simulink model "ModelMotorDiscreto"  (R2012b)
settings: Solver=ode4  StartTime=0.0  StopTime=15  FixedStep=1e-4  RelTol=1e-3
undefined symbols (not defined in the file or in its folder): C2t
libraries: simulink x2
settings Model: Creator=Augusto  LastModifiedBy=Augusto

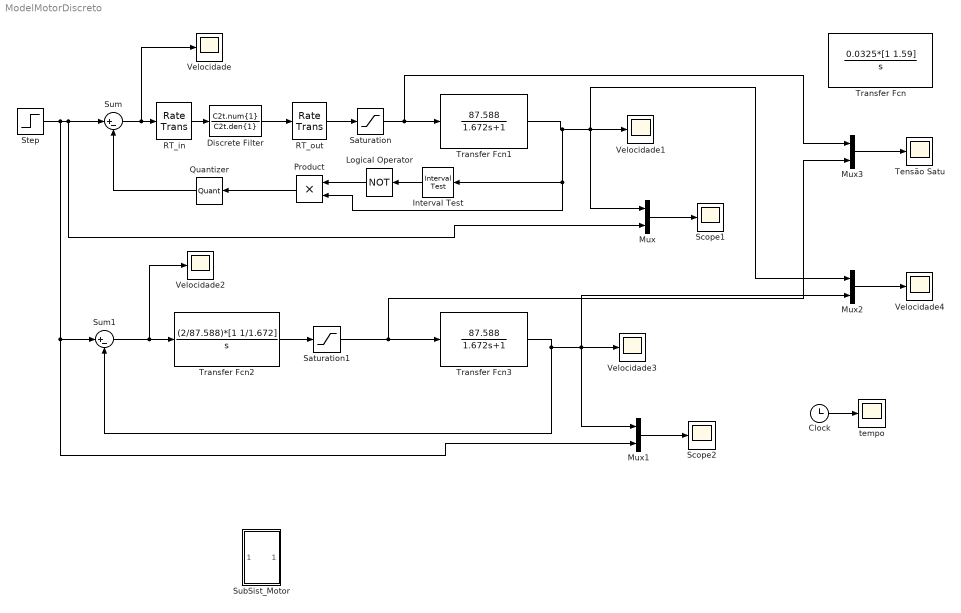
== system ModelMotorDiscreto ==
  Clock : Clock
  Discrete Filter : DiscreteFilter  Numerator=C2t.num{1}  Denominator=C2t.den{1}  SampleTime=C2t.Ts
  Interval Test : simulink/Logic and Bit Operations/Interval Test  IntervalClosedRight=on  uplimit=60*pi/30  IntervalClosedLeft=on  lowlimit=-60*pi/30  OutDataTypeStr=boolean
  Logical Operator : Logic  Operator=NOT  IconShape=distinctive  AllPortsSameDT=off  OutDataTypeStr=boolean
  Mux{,1..3} (4 alike) : Mux  Inputs=2
  Product : Product  RndMeth=Zero
  Quantizer : Quantizer  QuantizationInterval=100*pi/30
  RT_in : RateTransition  OutPortSampleTime=C2t.Ts
  RT_out : RateTransition  OutPortSampleTime=1e-4
  Saturation : Saturate  UpperLimit=11.4  LowerLimit=-11.4
  Saturation1 : Saturate  UpperLimit=11.4  LowerLimit=-11.4
  Scope1 : Scope
  Scope2 : Scope
      settings: YMin=628  YMax=628  SaveName=ScopeData3
  Step : Step  Time=100  Before=600  After=-628  SampleTime=0
  SubSist_Motor : Subsystem
  Sum : Sum  Inputs=|+-
  Sum1 : Sum  Inputs=|+-
  Tensão Satu : Scope
      settings: SaveName=ScopeData9
  Transfer Fcn : TransferFcn  Numerator=0.0325*[1 1.59]  Denominator=[1 0]
  Transfer Fcn1 : TransferFcn  Numerator=[87.588]  Denominator=[1.672 1]
  Transfer Fcn2 : TransferFcn  Numerator=(2/87.588)*[1 1/1.672]  Denominator=[1 0]
  Transfer Fcn3 : TransferFcn  Numerator=[87.588]  Denominator=[1.672 1]
  Velocidade{,1..4} (5 alike) : Scope
      Velocidade1 settings: SaveName=ScopeData2
      Velocidade2 settings: SaveName=ScopeData6
      Velocidade3 settings: SaveName=ScopeData7
      Velocidade4 settings: TimeRange=15  YMin=0  YMax=800  SaveName=ScopeData8
  tempo : Scope
      settings: Tag=Tempo  SaveName=ScopeData10
  wires:
  Mux/1 -> Scope1/1
  Sum/1 -> RT_in/1, Velocidade/1
  RT_out/1 -> Saturation/1
  Mux1/1 -> Scope2/1
  Sum1/1 -> Velocidade2/1, Transfer Fcn2/1
  Transfer Fcn2/1 -> Saturation1/1
  Transfer Fcn3/1 -> Sum1/2, Mux2/2, Mux1/1, Velocidade3/1
  Step/1 -> Sum1/1, Mux1/2, Sum/1, Mux/2
  Mux2/1 -> Velocidade4/1
  Saturation/1 -> Mux3/1, Transfer Fcn1/1
  Mux3/1 -> Tensão Satu/1
  Saturation1/1 -> Mux3/2, Transfer Fcn3/1
  Clock/1 -> tempo/1
  Discrete Filter/1 -> RT_out/1
  RT_in/1 -> Discrete Filter/1
  Transfer Fcn1/1 -> Interval Test/1, Product/2, Mux2/1, Mux/1, Velocidade1/1
  Product/1 -> Quantizer/1
  Interval Test/1 -> Logical Operator/1
  Logical Operator/1 -> Product/1
  Quantizer/1 -> Sum/2

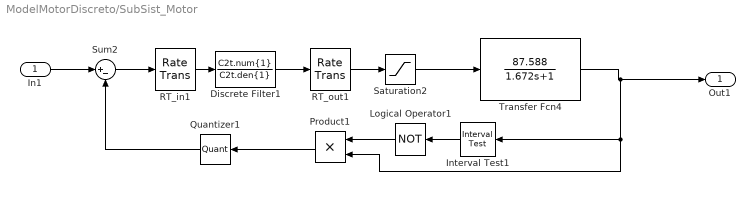
== system ModelMotorDiscreto/SubSist_Motor ==
  In1 : Inport
  Discrete Filter1 : DiscreteFilter  Numerator=C2t.num{1}  Denominator=C2t.den{1}  SampleTime=C2t.Ts
  Interval Test1 : simulink/Logic and Bit Operations/Interval Test  IntervalClosedRight=on  uplimit=60*pi/30  IntervalClosedLeft=on  lowlimit=-60*pi/30  OutDataTypeStr=boolean
  Logical Operator1 : Logic  Operator=NOT  IconShape=distinctive  AllPortsSameDT=off  OutDataTypeStr=boolean
  Product1 : Product  OutDataTypeStr=double  RndMeth=Zero
  Quantizer1 : Quantizer  QuantizationInterval=100*pi/30
  RT_in1 : RateTransition  OutPortSampleTime=C2t.Ts
  RT_out1 : RateTransition  OutPortSampleTime=1e-4
  Saturation2 : Saturate  UpperLimit=11.4  LowerLimit=-11.4
  Sum2 : Sum  Inputs=|+-
  Transfer Fcn4 : TransferFcn  Numerator=[87.588]  Denominator=[1.672 1]
  Out1 : Outport
  wires:
  Discrete Filter1/1 -> RT_out1/1
  RT_in1/1 -> Discrete Filter1/1
  Sum2/1 -> RT_in1/1
  In1/1 -> Sum2/1
  Saturation2/1 -> Transfer Fcn4/1
  RT_out1/1 -> Saturation2/1
  Transfer Fcn4/1 -> Out1/1, Interval Test1/1, Product1/2
  Product1/1 -> Quantizer1/1
  Interval Test1/1 -> Logical Operator1/1
  Logical Operator1/1 -> Product1/1
  Quantizer1/1 -> Sum2/2
